simulink subsystem "BatteryHVDetailed_refsub_MultiModule"  (R2022a)
settings: Solver=VariableStepAuto  StartTime=0.0  StopTime=10.0  RelTol=1e-3
undefined symbols (not defined in the file or in its folder): batteryHV_multi_pack1, batteryHV_multi_pack2
libraries: fl_lib x139, nesl_utility x29, batteryModule_lib x12
(part 3 of 3)

== system BatteryHVDetailed_refsub_MultiModule/BatteryPack1/negPlate_B14 ==
  Conductive Heat Transfer : fl_lib/Thermal/Thermal Elements/Conductive Heat Transfer  area=batteryHV_multi_pack1.batteryCell_H*batteryHV_multi_pack1.batteryCell_W m^2  thickness=0.002 m  th_cond=0.024 W/(m*K)  T_specify=off  T_priority=None  T=0 K  T_nominal_specify=off  T_nominal_unit=K  T_nominal_value=1  Q_specify=off  Q_priority=None  Q=0 W  Q_nominal_specify=off  Q_nominal_unit=W  Q_nominal_value=1
      settings: SourceProductBaseCode=PW,SS,VE
  Conductive Heat Transfer1 : fl_lib/Thermal/Thermal Elements/Conductive Heat Transfer  area=batteryHV_multi_pack1.batteryCell_H*batteryHV_multi_pack1.batteryCell_W m^2  thickness=0.002 m  th_cond=0.024 W/(m*K)  T_specify=off  T_priority=None  T=0 K  T_nominal_specify=off  T_nominal_unit=K  T_nominal_value=1  Q_specify=off  Q_priority=None  Q=0 W  Q_nominal_specify=off  Q_nominal_unit=W  Q_nominal_value=1
      settings: SourceProductBaseCode=PW,SS,VE
  plasticPlate : fl_lib/Thermal/Thermal Elements/Thermal Mass  mass=batteryHV_multi_pack1.batteryCell_H*batteryHV_multi_pack1.batteryCell_T*batteryHV_multi_pack1.battery_N_cells*0.002*44 kg  sp_heat=400 J/kg/K  T_specify=off  T_priority=High  T=300 K  T_nominal_specify=off  T_nominal_unit=K  T_nominal_value=1  Q_specify=off  Q_priority=None  Q=0 W  Q_nominal_specify=off  Q_nominal_unit=W  Q_nominal_value=1
      settings: SourceProductBaseCode=PW,SS,VE
  amb : PMIOPort  Side=Left
  M : PMIOPort  Port=2  Side=Right
  connections:
  Conductive Heat Transfer1/LConn1 -- Conductive Heat Transfer/RConn1 -- plasticPlate/LConn1
  Conductive Heat Transfer/LConn1 -- M/RConn1
  Conductive Heat Transfer1/RConn1 -- amb/RConn1

== system BatteryHVDetailed_refsub_MultiModule/BatteryPack1/negPlate_B16 ==
  Conductive Heat Transfer : fl_lib/Thermal/Thermal Elements/Conductive Heat Transfer  area=batteryHV_multi_pack1.batteryCell_H*batteryHV_multi_pack1.batteryCell_W m^2  thickness=0.002 m  th_cond=0.024 W/(m*K)  T_specify=off  T_priority=None  T=0 K  T_nominal_specify=off  T_nominal_unit=K  T_nominal_value=1  Q_specify=off  Q_priority=None  Q=0 W  Q_nominal_specify=off  Q_nominal_unit=W  Q_nominal_value=1
      settings: SourceProductBaseCode=PW,SS,VE
  Conductive Heat Transfer1 : fl_lib/Thermal/Thermal Elements/Conductive Heat Transfer  area=batteryHV_multi_pack1.batteryCell_H*batteryHV_multi_pack1.batteryCell_W m^2  thickness=0.002 m  th_cond=0.024 W/(m*K)  T_specify=off  T_priority=None  T=0 K  T_nominal_specify=off  T_nominal_unit=K  T_nominal_value=1  Q_specify=off  Q_priority=None  Q=0 W  Q_nominal_specify=off  Q_nominal_unit=W  Q_nominal_value=1
      settings: SourceProductBaseCode=PW,SS,VE
  plasticPlate : fl_lib/Thermal/Thermal Elements/Thermal Mass  mass=batteryHV_multi_pack1.batteryCell_H*batteryHV_multi_pack1.batteryCell_T*batteryHV_multi_pack1.battery_N_cells*0.002*44 kg  sp_heat=400 J/kg/K  T_specify=off  T_priority=High  T=300 K  T_nominal_specify=off  T_nominal_unit=K  T_nominal_value=1  Q_specify=off  Q_priority=None  Q=0 W  Q_nominal_specify=off  Q_nominal_unit=W  Q_nominal_value=1
      settings: SourceProductBaseCode=PW,SS,VE
  amb : PMIOPort  Side=Left
  M : PMIOPort  Port=2  Side=Right
  connections:
  Conductive Heat Transfer1/RConn1 -- amb/RConn1
  Conductive Heat Transfer/LConn1 -- M/RConn1
  plasticPlate/LConn1 -- Conductive Heat Transfer/RConn1 -- Conductive Heat Transfer1/LConn1

== system BatteryHVDetailed_refsub_MultiModule/BatteryPack1/posPlate_B11 ==
  Conductive Heat Transfer : fl_lib/Thermal/Thermal Elements/Conductive Heat Transfer  area=batteryHV_multi_pack1.batteryCell_H*batteryHV_multi_pack1.batteryCell_W m^2  thickness=0.002 m  th_cond=0.024 W/(m*K)  T_specify=off  T_priority=None  T=0 K  T_nominal_specify=off  T_nominal_unit=K  T_nominal_value=1  Q_specify=off  Q_priority=None  Q=0 W  Q_nominal_specify=off  Q_nominal_unit=W  Q_nominal_value=1
      settings: SourceProductBaseCode=PW,SS,VE
  Conductive Heat Transfer1 : fl_lib/Thermal/Thermal Elements/Conductive Heat Transfer  area=batteryHV_multi_pack1.batteryCell_H*batteryHV_multi_pack1.batteryCell_W m^2  thickness=0.002 m  th_cond=0.024 W/(m*K)  T_specify=off  T_priority=None  T=0 K  T_nominal_specify=off  T_nominal_unit=K  T_nominal_value=1  Q_specify=off  Q_priority=None  Q=0 W  Q_nominal_specify=off  Q_nominal_unit=W  Q_nominal_value=1
      settings: SourceProductBaseCode=PW,SS,VE
  plasticPlate : fl_lib/Thermal/Thermal Elements/Thermal Mass  mass=batteryHV_multi_pack1.batteryCell_H*batteryHV_multi_pack1.batteryCell_T*batteryHV_multi_pack1.battery_N_cells*0.002*44 kg  sp_heat=400 J/kg/K  T_specify=off  T_priority=High  T=300 K  T_nominal_specify=off  T_nominal_unit=K  T_nominal_value=1  Q_specify=off  Q_priority=None  Q=0 W  Q_nominal_specify=off  Q_nominal_unit=W  Q_nominal_value=1
      settings: SourceProductBaseCode=PW,SS,VE
  amb : PMIOPort  Side=Left
  M : PMIOPort  Port=2  Side=Right
  connections:
  Conductive Heat Transfer1/RConn1 -- amb/RConn1
  Conductive Heat Transfer/LConn1 -- M/RConn1
  plasticPlate/LConn1 -- Conductive Heat Transfer/RConn1 -- Conductive Heat Transfer1/LConn1

== system BatteryHVDetailed_refsub_MultiModule/BatteryPack1/posPlate_B13 ==
  Conductive Heat Transfer : fl_lib/Thermal/Thermal Elements/Conductive Heat Transfer  area=batteryHV_multi_pack1.batteryCell_H*batteryHV_multi_pack1.batteryCell_W m^2  thickness=0.002 m  th_cond=0.024 W/(m*K)  T_specify=off  T_priority=None  T=0 K  T_nominal_specify=off  T_nominal_unit=K  T_nominal_value=1  Q_specify=off  Q_priority=None  Q=0 W  Q_nominal_specify=off  Q_nominal_unit=W  Q_nominal_value=1
      settings: SourceProductBaseCode=PW,SS,VE
  Conductive Heat Transfer1 : fl_lib/Thermal/Thermal Elements/Conductive Heat Transfer  area=batteryHV_multi_pack1.batteryCell_H*batteryHV_multi_pack1.batteryCell_W m^2  thickness=0.002 m  th_cond=0.024 W/(m*K)  T_specify=off  T_priority=None  T=0 K  T_nominal_specify=off  T_nominal_unit=K  T_nominal_value=1  Q_specify=off  Q_priority=None  Q=0 W  Q_nominal_specify=off  Q_nominal_unit=W  Q_nominal_value=1
      settings: SourceProductBaseCode=PW,SS,VE
  plasticPlate : fl_lib/Thermal/Thermal Elements/Thermal Mass  mass=batteryHV_multi_pack1.batteryCell_H*batteryHV_multi_pack1.batteryCell_T*batteryHV_multi_pack1.battery_N_cells*0.002*44 kg  sp_heat=400 J/kg/K  T_specify=off  T_priority=High  T=300 K  T_nominal_specify=off  T_nominal_unit=K  T_nominal_value=1  Q_specify=off  Q_priority=None  Q=0 W  Q_nominal_specify=off  Q_nominal_unit=W  Q_nominal_value=1
      settings: SourceProductBaseCode=PW,SS,VE
  amb : PMIOPort  Side=Left
  M : PMIOPort  Port=2  Side=Right
  connections:
  Conductive Heat Transfer1/RConn1 -- amb/RConn1
  Conductive Heat Transfer/LConn1 -- M/RConn1
  plasticPlate/LConn1 -- Conductive Heat Transfer/RConn1 -- Conductive Heat Transfer1/LConn1

== system BatteryHVDetailed_refsub_MultiModule/BatteryPack1/posPlate_B15 ==
  Conductive Heat Transfer : fl_lib/Thermal/Thermal Elements/Conductive Heat Transfer  area=batteryHV_multi_pack1.batteryCell_H*batteryHV_multi_pack1.batteryCell_W m^2  thickness=0.002 m  th_cond=0.024 W/(m*K)  T_specify=off  T_priority=None  T=0 K  T_nominal_specify=off  T_nominal_unit=K  T_nominal_value=1  Q_specify=off  Q_priority=None  Q=0 W  Q_nominal_specify=off  Q_nominal_unit=W  Q_nominal_value=1
      settings: SourceProductBaseCode=PW,SS,VE
  Conductive Heat Transfer1 : fl_lib/Thermal/Thermal Elements/Conductive Heat Transfer  area=batteryHV_multi_pack1.batteryCell_H*batteryHV_multi_pack1.batteryCell_W m^2  thickness=0.002 m  th_cond=0.024 W/(m*K)  T_specify=off  T_priority=None  T=0 K  T_nominal_specify=off  T_nominal_unit=K  T_nominal_value=1  Q_specify=off  Q_priority=None  Q=0 W  Q_nominal_specify=off  Q_nominal_unit=W  Q_nominal_value=1
      settings: SourceProductBaseCode=PW,SS,VE
  plasticPlate : fl_lib/Thermal/Thermal Elements/Thermal Mass  mass=batteryHV_multi_pack1.batteryCell_H*batteryHV_multi_pack1.batteryCell_T*batteryHV_multi_pack1.battery_N_cells*0.002*44 kg  sp_heat=400 J/kg/K  T_specify=off  T_priority=High  T=300 K  T_nominal_specify=off  T_nominal_unit=K  T_nominal_value=1  Q_specify=off  Q_priority=None  Q=0 W  Q_nominal_specify=off  Q_nominal_unit=W  Q_nominal_value=1
      settings: SourceProductBaseCode=PW,SS,VE
  amb : PMIOPort  Side=Left
  M : PMIOPort  Port=2  Side=Right
  connections:
  Conductive Heat Transfer1/LConn1 -- Conductive Heat Transfer/RConn1 -- plasticPlate/LConn1
  Conductive Heat Transfer/LConn1 -- M/RConn1
  Conductive Heat Transfer1/RConn1 -- amb/RConn1

== system BatteryHVDetailed_refsub_MultiModule/BatteryPack1/rightPlate_B15 ==
  Conductive Heat Transfer : fl_lib/Thermal/Thermal Elements/Conductive Heat Transfer  area=batteryHV_multi_pack1.batteryCell_H*batteryHV_multi_pack1.batteryCell_T*batteryHV_multi_pack1.battery_N_cells m^2  thickness=0.002 m  th_cond=0.024 W/(m*K)  T_specify=off  T_priority=None  T=0 K  T_nominal_specify=off  T_nominal_unit=K  T_nominal_value=1  Q_specify=off  Q_priority=None  Q=0 W  Q_nominal_specify=off  Q_nominal_unit=W  Q_nominal_value=1
      settings: SourceProductBaseCode=PW,SS,VE
  Conductive Heat Transfer1 : fl_lib/Thermal/Thermal Elements/Conductive Heat Transfer  area=batteryHV_multi_pack1.batteryCell_H*batteryHV_multi_pack1.batteryCell_T*batteryHV_multi_pack1.battery_N_cells m^2  thickness=0.002 m  th_cond=0.024 W/(m*K)  T_specify=off  T_priority=None  T=0 K  T_nominal_specify=off  T_nominal_unit=K  T_nominal_value=1  Q_specify=off  Q_priority=None  Q=0 W  Q_nominal_specify=off  Q_nominal_unit=W  Q_nominal_value=1
      settings: SourceProductBaseCode=PW,SS,VE
  plasticPlate : fl_lib/Thermal/Thermal Elements/Thermal Mass  mass=batteryHV_multi_pack1.batteryCell_H*batteryHV_multi_pack1.batteryCell_T*batteryHV_multi_pack1.battery_N_cells*0.002*44 kg  sp_heat=400 J/kg/K  T_specify=off  T_priority=High  T=300 K  T_nominal_specify=off  T_nominal_unit=K  T_nominal_value=1  Q_specify=off  Q_priority=None  Q=0 W  Q_nominal_specify=off  Q_nominal_unit=W  Q_nominal_value=1
      settings: SourceProductBaseCode=PW,SS,VE
  amb : PMIOPort  Side=Left
  M : PMIOPort  Port=2  Side=Right
  connections:
  Conductive Heat Transfer1/RConn1 -- amb/RConn1
  Conductive Heat Transfer/LConn1 -- M/RConn1
  plasticPlate/LConn1 -- Conductive Heat Transfer/RConn1 -- Conductive Heat Transfer1/LConn1

== system BatteryHVDetailed_refsub_MultiModule/BatteryPack1/rightPlate_B16 ==
  Conductive Heat Transfer : fl_lib/Thermal/Thermal Elements/Conductive Heat Transfer  area=batteryHV_multi_pack1.batteryCell_H*batteryHV_multi_pack1.batteryCell_T*batteryHV_multi_pack1.battery_N_cells m^2  thickness=0.002 m  th_cond=0.024 W/(m*K)  T_specify=off  T_priority=None  T=0 K  T_nominal_specify=off  T_nominal_unit=K  T_nominal_value=1  Q_specify=off  Q_priority=None  Q=0 W  Q_nominal_specify=off  Q_nominal_unit=W  Q_nominal_value=1
      settings: SourceProductBaseCode=PW,SS,VE
  Conductive Heat Transfer1 : fl_lib/Thermal/Thermal Elements/Conductive Heat Transfer  area=batteryHV_multi_pack1.batteryCell_H*batteryHV_multi_pack1.batteryCell_T*batteryHV_multi_pack1.battery_N_cells m^2  thickness=0.002 m  th_cond=0.024 W/(m*K)  T_specify=off  T_priority=None  T=0 K  T_nominal_specify=off  T_nominal_unit=K  T_nominal_value=1  Q_specify=off  Q_priority=None  Q=0 W  Q_nominal_specify=off  Q_nominal_unit=W  Q_nominal_value=1
      settings: SourceProductBaseCode=PW,SS,VE
  plasticPlate : fl_lib/Thermal/Thermal Elements/Thermal Mass  mass=batteryHV_multi_pack1.batteryCell_H*batteryHV_multi_pack1.batteryCell_T*batteryHV_multi_pack1.battery_N_cells*0.002*44 kg  sp_heat=400 J/kg/K  T_specify=off  T_priority=High  T=300 K  T_nominal_specify=off  T_nominal_unit=K  T_nominal_value=1  Q_specify=off  Q_priority=None  Q=0 W  Q_nominal_specify=off  Q_nominal_unit=W  Q_nominal_value=1
      settings: SourceProductBaseCode=PW,SS,VE
  amb : PMIOPort  Side=Left
  M : PMIOPort  Port=2  Side=Right
  connections:
  Conductive Heat Transfer1/LConn1 -- Conductive Heat Transfer/RConn1 -- plasticPlate/LConn1
  Conductive Heat Transfer/LConn1 -- M/RConn1
  Conductive Heat Transfer1/RConn1 -- amb/RConn1

== system BatteryHVDetailed_refsub_MultiModule/BatteryPack2/air gap 2-1 ==
  Conductive Heat Transfer : fl_lib/Thermal/Thermal Elements/Conductive Heat Transfer  area=batteryHV_multi_pack1.batteryCell_T*batteryHV_multi_pack1.battery_N_cells*batteryHV_multi_pack1.batteryCell_H m^2  thickness=0.002 m  th_cond=0.024 W/(m*K)  T_specify=off  T_priority=None  T=0 K  T_nominal_specify=off  T_nominal_unit=K  T_nominal_value=1  Q_specify=off  Q_priority=None  Q=0 W  Q_nominal_specify=off  Q_nominal_unit=W  Q_nominal_value=1
      settings: SourceProductBaseCode=PW,SS,VE
  Conductive Heat Transfer1 : fl_lib/Thermal/Thermal Elements/Conductive Heat Transfer  area=batteryHV_multi_pack1.batteryCell_H*batteryHV_multi_pack1.batteryCell_H m^2  thickness=0.002 m  th_cond=0.024 W/(m*K)  T_specify=off  T_priority=None  T=0 K  T_nominal_specify=off  T_nominal_unit=K  T_nominal_value=1  Q_specify=off  Q_priority=None  Q=0 W  Q_nominal_specify=off  Q_nominal_unit=W  Q_nominal_value=1
      settings: SourceProductBaseCode=PW,SS,VE
  air mass : fl_lib/Thermal/Thermal Elements/Thermal Mass  mass=batteryHV_multi_pack1.batteryCell_H*batteryHV_multi_pack1.batteryCell_T*batteryHV_multi_pack1.battery_N_cells*0.002*1.28 kg  sp_heat=1000 J/kg/K  T_specify=off  T_priority=High  T=300 K  T_nominal_specify=off  T_nominal_unit=K  T_nominal_value=1  Q_specify=off  Q_priority=None  Q=0 W  Q_nominal_specify=off  Q_nominal_unit=W  Q_nominal_value=1
      settings: SourceProductBaseCode=PW,SS,VE
  M2 : PMIOPort  Side=Left
  M1 : PMIOPort  Port=2  Side=Right
  connections:
  Conductive Heat Transfer1/LConn1 -- Conductive Heat Transfer/RConn1 -- air mass/LConn1
  Conductive Heat Transfer1/RConn1 -- M1/RConn1
  Conductive Heat Transfer/LConn1 -- M2/RConn1

== system BatteryHVDetailed_refsub_MultiModule/BatteryPack2/air gap 3-2 ==
  Conductive Heat Transfer : fl_lib/Thermal/Thermal Elements/Conductive Heat Transfer  area=batteryHV_multi_pack1.batteryCell_T*batteryHV_multi_pack1.battery_N_cells*batteryHV_multi_pack1.batteryCell_H m^2  thickness=0.002 m  th_cond=0.024 W/(m*K)  T_specify=off  T_priority=None  T=0 K  T_nominal_specify=off  T_nominal_unit=K  T_nominal_value=1  Q_specify=off  Q_priority=None  Q=0 W  Q_nominal_specify=off  Q_nominal_unit=W  Q_nominal_value=1
      settings: SourceProductBaseCode=PW,SS,VE
  Conductive Heat Transfer1 : fl_lib/Thermal/Thermal Elements/Conductive Heat Transfer  area=batteryHV_multi_pack1.batteryCell_H*batteryHV_multi_pack1.batteryCell_H m^2  thickness=0.002 m  th_cond=0.024 W/(m*K)  T_specify=off  T_priority=None  T=0 K  T_nominal_specify=off  T_nominal_unit=K  T_nominal_value=1  Q_specify=off  Q_priority=None  Q=0 W  Q_nominal_specify=off  Q_nominal_unit=W  Q_nominal_value=1
      settings: SourceProductBaseCode=PW,SS,VE
  air mass : fl_lib/Thermal/Thermal Elements/Thermal Mass  mass=batteryHV_multi_pack1.batteryCell_H*batteryHV_multi_pack1.batteryCell_T*batteryHV_multi_pack1.battery_N_cells*0.002*1.28 kg  sp_heat=1000 J/kg/K  T_specify=off  T_priority=High  T=300 K  T_nominal_specify=off  T_nominal_unit=K  T_nominal_value=1  Q_specify=off  Q_priority=None  Q=0 W  Q_nominal_specify=off  Q_nominal_unit=W  Q_nominal_value=1
      settings: SourceProductBaseCode=PW,SS,VE
  M3 : PMIOPort  Side=Left
  M2 : PMIOPort  Port=2  Side=Right
  connections:
  Conductive Heat Transfer/LConn1 -- M3/RConn1
  Conductive Heat Transfer1/RConn1 -- M2/RConn1
  air mass/LConn1 -- Conductive Heat Transfer/RConn1 -- Conductive Heat Transfer1/LConn1

== system BatteryHVDetailed_refsub_MultiModule/BatteryPack2/air gap 4-3 ==
  Conductive Heat Transfer : fl_lib/Thermal/Thermal Elements/Conductive Heat Transfer  area=batteryHV_multi_pack1.batteryCell_T*batteryHV_multi_pack1.battery_N_cells*batteryHV_multi_pack1.batteryCell_H m^2  thickness=0.002 m  th_cond=0.024 W/(m*K)  T_specify=off  T_priority=None  T=0 K  T_nominal_specify=off  T_nominal_unit=K  T_nominal_value=1  Q_specify=off  Q_priority=None  Q=0 W  Q_nominal_specify=off  Q_nominal_unit=W  Q_nominal_value=1
      settings: SourceProductBaseCode=PW,SS,VE
  Conductive Heat Transfer1 : fl_lib/Thermal/Thermal Elements/Conductive Heat Transfer  area=batteryHV_multi_pack1.batteryCell_H*batteryHV_multi_pack1.batteryCell_H m^2  thickness=0.002 m  th_cond=0.024 W/(m*K)  T_specify=off  T_priority=None  T=0 K  T_nominal_specify=off  T_nominal_unit=K  T_nominal_value=1  Q_specify=off  Q_priority=None  Q=0 W  Q_nominal_specify=off  Q_nominal_unit=W  Q_nominal_value=1
      settings: SourceProductBaseCode=PW,SS,VE
  air mass : fl_lib/Thermal/Thermal Elements/Thermal Mass  mass=batteryHV_multi_pack1.batteryCell_H*batteryHV_multi_pack1.batteryCell_T*batteryHV_multi_pack1.battery_N_cells*0.002*1.28 kg  sp_heat=1000 J/kg/K  T_specify=off  T_priority=High  T=300 K  T_nominal_specify=off  T_nominal_unit=K  T_nominal_value=1  Q_specify=off  Q_priority=None  Q=0 W  Q_nominal_specify=off  Q_nominal_unit=W  Q_nominal_value=1
      settings: SourceProductBaseCode=PW,SS,VE
  M4 : PMIOPort  Side=Left
  M3 : PMIOPort  Port=2  Side=Right
  connections:
  Conductive Heat Transfer1/LConn1 -- Conductive Heat Transfer/RConn1 -- air mass/LConn1
  Conductive Heat Transfer1/RConn1 -- M3/RConn1
  Conductive Heat Transfer/LConn1 -- M4/RConn1

== system BatteryHVDetailed_refsub_MultiModule/BatteryPack2/air gap 5-4 ==
  Conductive Heat Transfer : fl_lib/Thermal/Thermal Elements/Conductive Heat Transfer  area=batteryHV_multi_pack1.batteryCell_T*batteryHV_multi_pack1.battery_N_cells*batteryHV_multi_pack1.batteryCell_H m^2  thickness=0.002 m  th_cond=0.024 W/(m*K)  T_specify=off  T_priority=None  T=0 K  T_nominal_specify=off  T_nominal_unit=K  T_nominal_value=1  Q_specify=off  Q_priority=None  Q=0 W  Q_nominal_specify=off  Q_nominal_unit=W  Q_nominal_value=1
      settings: SourceProductBaseCode=PW,SS,VE
  Conductive Heat Transfer1 : fl_lib/Thermal/Thermal Elements/Conductive Heat Transfer  area=batteryHV_multi_pack1.batteryCell_H*batteryHV_multi_pack1.batteryCell_H m^2  thickness=0.002 m  th_cond=0.024 W/(m*K)  T_specify=off  T_priority=None  T=0 K  T_nominal_specify=off  T_nominal_unit=K  T_nominal_value=1  Q_specify=off  Q_priority=None  Q=0 W  Q_nominal_specify=off  Q_nominal_unit=W  Q_nominal_value=1
      settings: SourceProductBaseCode=PW,SS,VE
  air mass : fl_lib/Thermal/Thermal Elements/Thermal Mass  mass=batteryHV_multi_pack1.batteryCell_H*batteryHV_multi_pack1.batteryCell_T*batteryHV_multi_pack1.battery_N_cells*0.002*1.28 kg  sp_heat=1000 J/kg/K  T_specify=off  T_priority=High  T=300 K  T_nominal_specify=off  T_nominal_unit=K  T_nominal_value=1  Q_specify=off  Q_priority=None  Q=0 W  Q_nominal_specify=off  Q_nominal_unit=W  Q_nominal_value=1
      settings: SourceProductBaseCode=PW,SS,VE
  M5 : PMIOPort  Side=Left
  M4 : PMIOPort  Port=2  Side=Right
  connections:
  Conductive Heat Transfer/LConn1 -- M5/RConn1
  Conductive Heat Transfer1/RConn1 -- M4/RConn1
  air mass/LConn1 -- Conductive Heat Transfer/RConn1 -- Conductive Heat Transfer1/LConn1

== system BatteryHVDetailed_refsub_MultiModule/BatteryPack2/air gap 5-6 ==
  Conductive Heat Transfer : fl_lib/Thermal/Thermal Elements/Conductive Heat Transfer  area=batteryHV_multi_pack2.batteryCell_T*batteryHV_multi_pack2.battery_N_cells*batteryHV_multi_pack2.batteryCell_W m^2  thickness=0.002 m  th_cond=0.024 W/(m*K)  T_specify=off  T_priority=None  T=0 K  T_nominal_specify=off  T_nominal_unit=K  T_nominal_value=1  Q_specify=off  Q_priority=None  Q=0 W  Q_nominal_specify=off  Q_nominal_unit=W  Q_nominal_value=1
      settings: SourceProductBaseCode=PW,SS,VE
  Conductive Heat Transfer1 : fl_lib/Thermal/Thermal Elements/Conductive Heat Transfer  area=batteryHV_multi_pack2.batteryCell_H*batteryHV_multi_pack2.batteryCell_W m^2  thickness=0.002 m  th_cond=0.024 W/(m*K)  T_specify=off  T_priority=None  T=0 K  T_nominal_specify=off  T_nominal_unit=K  T_nominal_value=1  Q_specify=off  Q_priority=None  Q=0 W  Q_nominal_specify=off  Q_nominal_unit=W  Q_nominal_value=1
      settings: SourceProductBaseCode=PW,SS,VE
  air mass : fl_lib/Thermal/Thermal Elements/Thermal Mass  mass=batteryHV_multi_pack2.batteryCell_W*batteryHV_multi_pack2.batteryCell_T*batteryHV_multi_pack2.battery_N_cells*0.002*1.28 kg  sp_heat=1000 J/kg/K  T_specify=off  T_priority=High  T=300 K  T_nominal_specify=off  T_nominal_unit=K  T_nominal_value=1  Q_specify=off  Q_priority=None  Q=0 W  Q_nominal_specify=off  Q_nominal_unit=W  Q_nominal_value=1
      settings: SourceProductBaseCode=PW,SS,VE
  M5 : PMIOPort  Side=Left
  M6 : PMIOPort  Port=2  Side=Right
  connections:
  Conductive Heat Transfer/LConn1 -- M5/RConn1
  Conductive Heat Transfer1/RConn1 -- M6/RConn1
  air mass/LConn1 -- Conductive Heat Transfer/RConn1 -- Conductive Heat Transfer1/LConn1

== system BatteryHVDetailed_refsub_MultiModule/BatteryPack2/leftPlate_B11 ==
  Conductive Heat Transfer : fl_lib/Thermal/Thermal Elements/Conductive Heat Transfer  area=batteryHV_multi_pack2.batteryCell_H*batteryHV_multi_pack2.batteryCell_T*batteryHV_multi_pack2.battery_N_cells m^2  thickness=0.002 m  th_cond=0.024 W/(m*K)  T_specify=off  T_priority=None  T=0 K  T_nominal_specify=off  T_nominal_unit=K  T_nominal_value=1  Q_specify=off  Q_priority=None  Q=0 W  Q_nominal_specify=off  Q_nominal_unit=W  Q_nominal_value=1
      settings: SourceProductBaseCode=PW,SS,VE
  Conductive Heat Transfer1 : fl_lib/Thermal/Thermal Elements/Conductive Heat Transfer  area=batteryHV_multi_pack2.batteryCell_H*batteryHV_multi_pack2.batteryCell_T*batteryHV_multi_pack2.battery_N_cells m^2  thickness=0.002 m  th_cond=0.024 W/(m*K)  T_specify=off  T_priority=None  T=0 K  T_nominal_specify=off  T_nominal_unit=K  T_nominal_value=1  Q_specify=off  Q_priority=None  Q=0 W  Q_nominal_specify=off  Q_nominal_unit=W  Q_nominal_value=1
      settings: SourceProductBaseCode=PW,SS,VE
  plasticPlate : fl_lib/Thermal/Thermal Elements/Thermal Mass  mass=batteryHV_multi_pack2.batteryCell_H*batteryHV_multi_pack2.batteryCell_T*batteryHV_multi_pack2.battery_N_cells*0.002*44 kg  sp_heat=400 J/kg/K  T_specify=off  T_priority=High  T=300 K  T_nominal_specify=off  T_nominal_unit=K  T_nominal_value=1  Q_specify=off  Q_priority=None  Q=0 W  Q_nominal_specify=off  Q_nominal_unit=W  Q_nominal_value=1
      settings: SourceProductBaseCode=PW,SS,VE
  amb : PMIOPort  Side=Left
  M : PMIOPort  Port=2  Side=Right
  connections:
  Conductive Heat Transfer1/LConn1 -- Conductive Heat Transfer/RConn1 -- plasticPlate/LConn1
  Conductive Heat Transfer/LConn1 -- M/RConn1
  Conductive Heat Transfer1/RConn1 -- amb/RConn1

== system BatteryHVDetailed_refsub_MultiModule/BatteryPack2/leftPlate_B16 ==
  Conductive Heat Transfer : fl_lib/Thermal/Thermal Elements/Conductive Heat Transfer  area=batteryHV_multi_pack2.batteryCell_H*batteryHV_multi_pack2.batteryCell_T*batteryHV_multi_pack2.battery_N_cells m^2  thickness=0.002 m  th_cond=0.024 W/(m*K)  T_specify=off  T_priority=None  T=0 K  T_nominal_specify=off  T_nominal_unit=K  T_nominal_value=1  Q_specify=off  Q_priority=None  Q=0 W  Q_nominal_specify=off  Q_nominal_unit=W  Q_nominal_value=1
      settings: SourceProductBaseCode=PW,SS,VE
  Conductive Heat Transfer1 : fl_lib/Thermal/Thermal Elements/Conductive Heat Transfer  area=batteryHV_multi_pack2.batteryCell_H*batteryHV_multi_pack2.batteryCell_T*batteryHV_multi_pack2.battery_N_cells m^2  thickness=0.002 m  th_cond=0.024 W/(m*K)  T_specify=off  T_priority=None  T=0 K  T_nominal_specify=off  T_nominal_unit=K  T_nominal_value=1  Q_specify=off  Q_priority=None  Q=0 W  Q_nominal_specify=off  Q_nominal_unit=W  Q_nominal_value=1
      settings: SourceProductBaseCode=PW,SS,VE
  plasticPlate : fl_lib/Thermal/Thermal Elements/Thermal Mass  mass=batteryHV_multi_pack2.batteryCell_H*batteryHV_multi_pack2.batteryCell_T*batteryHV_multi_pack2.battery_N_cells*0.002*44 kg  sp_heat=400 J/kg/K  T_specify=off  T_priority=High  T=300 K  T_nominal_specify=off  T_nominal_unit=K  T_nominal_value=1  Q_specify=off  Q_priority=None  Q=0 W  Q_nominal_specify=off  Q_nominal_unit=W  Q_nominal_value=1
      settings: SourceProductBaseCode=PW,SS,VE
  amb : PMIOPort  Side=Left
  M : PMIOPort  Port=2  Side=Right
  connections:
  Conductive Heat Transfer1/LConn1 -- Conductive Heat Transfer/RConn1 -- plasticPlate/LConn1
  Conductive Heat Transfer/LConn1 -- M/RConn1
  Conductive Heat Transfer1/RConn1 -- amb/RConn1

== system BatteryHVDetailed_refsub_MultiModule/BatteryPack2/negPlate_B12 ==
  Conductive Heat Transfer : fl_lib/Thermal/Thermal Elements/Conductive Heat Transfer  area=batteryHV_multi_pack2.batteryCell_H*batteryHV_multi_pack2.batteryCell_W m^2  thickness=0.002 m  th_cond=0.024 W/(m*K)  T_specify=off  T_priority=None  T=0 K  T_nominal_specify=off  T_nominal_unit=K  T_nominal_value=1  Q_specify=off  Q_priority=None  Q=0 W  Q_nominal_specify=off  Q_nominal_unit=W  Q_nominal_value=1
      settings: SourceProductBaseCode=PW,SS,VE
  Conductive Heat Transfer1 : fl_lib/Thermal/Thermal Elements/Conductive Heat Transfer  area=batteryHV_multi_pack2.batteryCell_H*batteryHV_multi_pack2.batteryCell_W m^2  thickness=0.002 m  th_cond=0.024 W/(m*K)  T_specify=off  T_priority=None  T=0 K  T_nominal_specify=off  T_nominal_unit=K  T_nominal_value=1  Q_specify=off  Q_priority=None  Q=0 W  Q_nominal_specify=off  Q_nominal_unit=W  Q_nominal_value=1
      settings: SourceProductBaseCode=PW,SS,VE
  plasticPlate : fl_lib/Thermal/Thermal Elements/Thermal Mass  mass=batteryHV_multi_pack2.batteryCell_H*batteryHV_multi_pack2.batteryCell_T*batteryHV_multi_pack2.battery_N_cells*0.002*44 kg  sp_heat=400 J/kg/K  T_specify=off  T_priority=High  T=300 K  T_nominal_specify=off  T_nominal_unit=K  T_nominal_value=1  Q_specify=off  Q_priority=None  Q=0 W  Q_nominal_specify=off  Q_nominal_unit=W  Q_nominal_value=1
      settings: SourceProductBaseCode=PW,SS,VE
  amb : PMIOPort  Side=Left
  M : PMIOPort  Port=2  Side=Right
  connections:
  Conductive Heat Transfer1/RConn1 -- amb/RConn1
  Conductive Heat Transfer/LConn1 -- M/RConn1
  plasticPlate/LConn1 -- Conductive Heat Transfer/RConn1 -- Conductive Heat Transfer1/LConn1

== system BatteryHVDetailed_refsub_MultiModule/BatteryPack2/negPlate_B14 ==
  Conductive Heat Transfer : fl_lib/Thermal/Thermal Elements/Conductive Heat Transfer  area=batteryHV_multi_pack2.batteryCell_H*batteryHV_multi_pack2.batteryCell_W m^2  thickness=0.002 m  th_cond=0.024 W/(m*K)  T_specify=off  T_priority=None  T=0 K  T_nominal_specify=off  T_nominal_unit=K  T_nominal_value=1  Q_specify=off  Q_priority=None  Q=0 W  Q_nominal_specify=off  Q_nominal_unit=W  Q_nominal_value=1
      settings: SourceProductBaseCode=PW,SS,VE
  Conductive Heat Transfer1 : fl_lib/Thermal/Thermal Elements/Conductive Heat Transfer  area=batteryHV_multi_pack2.batteryCell_H*batteryHV_multi_pack2.batteryCell_W m^2  thickness=0.002 m  th_cond=0.024 W/(m*K)  T_specify=off  T_priority=None  T=0 K  T_nominal_specify=off  T_nominal_unit=K  T_nominal_value=1  Q_specify=off  Q_priority=None  Q=0 W  Q_nominal_specify=off  Q_nominal_unit=W  Q_nominal_value=1
      settings: SourceProductBaseCode=PW,SS,VE
  plasticPlate : fl_lib/Thermal/Thermal Elements/Thermal Mass  mass=batteryHV_multi_pack2.batteryCell_H*batteryHV_multi_pack2.batteryCell_T*batteryHV_multi_pack2.battery_N_cells*0.002*44 kg  sp_heat=400 J/kg/K  T_specify=off  T_priority=High  T=300 K  T_nominal_specify=off  T_nominal_unit=K  T_nominal_value=1  Q_specify=off  Q_priority=None  Q=0 W  Q_nominal_specify=off  Q_nominal_unit=W  Q_nominal_value=1
      settings: SourceProductBaseCode=PW,SS,VE
  amb : PMIOPort  Side=Left
  M : PMIOPort  Port=2  Side=Right
  connections:
  Conductive Heat Transfer1/RConn1 -- amb/RConn1
  Conductive Heat Transfer/LConn1 -- M/RConn1
  plasticPlate/LConn1 -- Conductive Heat Transfer/RConn1 -- Conductive Heat Transfer1/LConn1

== system BatteryHVDetailed_refsub_MultiModule/BatteryPack2/negPlate_B16 ==
  Conductive Heat Transfer : fl_lib/Thermal/Thermal Elements/Conductive Heat Transfer  area=batteryHV_multi_pack2.batteryCell_H*batteryHV_multi_pack2.batteryCell_W m^2  thickness=0.002 m  th_cond=0.024 W/(m*K)  T_specify=off  T_priority=None  T=0 K  T_nominal_specify=off  T_nominal_unit=K  T_nominal_value=1  Q_specify=off  Q_priority=None  Q=0 W  Q_nominal_specify=off  Q_nominal_unit=W  Q_nominal_value=1
      settings: SourceProductBaseCode=PW,SS,VE
  Conductive Heat Transfer1 : fl_lib/Thermal/Thermal Elements/Conductive Heat Transfer  area=batteryHV_multi_pack2.batteryCell_H*batteryHV_multi_pack2.batteryCell_W m^2  thickness=0.002 m  th_cond=0.024 W/(m*K)  T_specify=off  T_priority=None  T=0 K  T_nominal_specify=off  T_nominal_unit=K  T_nominal_value=1  Q_specify=off  Q_priority=None  Q=0 W  Q_nominal_specify=off  Q_nominal_unit=W  Q_nominal_value=1
      settings: SourceProductBaseCode=PW,SS,VE
  plasticPlate : fl_lib/Thermal/Thermal Elements/Thermal Mass  mass=batteryHV_multi_pack2.batteryCell_H*batteryHV_multi_pack2.batteryCell_T*batteryHV_multi_pack2.battery_N_cells*0.002*44 kg  sp_heat=400 J/kg/K  T_specify=off  T_priority=High  T=300 K  T_nominal_specify=off  T_nominal_unit=K  T_nominal_value=1  Q_specify=off  Q_priority=None  Q=0 W  Q_nominal_specify=off  Q_nominal_unit=W  Q_nominal_value=1
      settings: SourceProductBaseCode=PW,SS,VE
  amb : PMIOPort  Side=Left
  M : PMIOPort  Port=2  Side=Right
  connections:
  Conductive Heat Transfer1/LConn1 -- Conductive Heat Transfer/RConn1 -- plasticPlate/LConn1
  Conductive Heat Transfer/LConn1 -- M/RConn1
  Conductive Heat Transfer1/RConn1 -- amb/RConn1

== system BatteryHVDetailed_refsub_MultiModule/BatteryPack2/posPlate_B11 ==
  Conductive Heat Transfer : fl_lib/Thermal/Thermal Elements/Conductive Heat Transfer  area=batteryHV_multi_pack2.batteryCell_H*batteryHV_multi_pack2.batteryCell_W m^2  thickness=0.002 m  th_cond=0.024 W/(m*K)  T_specify=off  T_priority=None  T=0 K  T_nominal_specify=off  T_nominal_unit=K  T_nominal_value=1  Q_specify=off  Q_priority=None  Q=0 W  Q_nominal_specify=off  Q_nominal_unit=W  Q_nominal_value=1
      settings: SourceProductBaseCode=PW,SS,VE
  Conductive Heat Transfer1 : fl_lib/Thermal/Thermal Elements/Conductive Heat Transfer  area=batteryHV_multi_pack2.batteryCell_H*batteryHV_multi_pack2.batteryCell_W m^2  thickness=0.002 m  th_cond=0.024 W/(m*K)  T_specify=off  T_priority=None  T=0 K  T_nominal_specify=off  T_nominal_unit=K  T_nominal_value=1  Q_specify=off  Q_priority=None  Q=0 W  Q_nominal_specify=off  Q_nominal_unit=W  Q_nominal_value=1
      settings: SourceProductBaseCode=PW,SS,VE
  plasticPlate : fl_lib/Thermal/Thermal Elements/Thermal Mass  mass=batteryHV_multi_pack2.batteryCell_H*batteryHV_multi_pack2.batteryCell_T*batteryHV_multi_pack2.battery_N_cells*0.002*44 kg  sp_heat=400 J/kg/K  T_specify=off  T_priority=High  T=300 K  T_nominal_specify=off  T_nominal_unit=K  T_nominal_value=1  Q_specify=off  Q_priority=None  Q=0 W  Q_nominal_specify=off  Q_nominal_unit=W  Q_nominal_value=1
      settings: SourceProductBaseCode=PW,SS,VE
  amb : PMIOPort  Side=Left
  M : PMIOPort  Port=2  Side=Right
  connections:
  Conductive Heat Transfer1/LConn1 -- Conductive Heat Transfer/RConn1 -- plasticPlate/LConn1
  Conductive Heat Transfer/LConn1 -- M/RConn1
  Conductive Heat Transfer1/RConn1 -- amb/RConn1

== system BatteryHVDetailed_refsub_MultiModule/BatteryPack2/posPlate_B13 ==
  Conductive Heat Transfer : fl_lib/Thermal/Thermal Elements/Conductive Heat Transfer  area=batteryHV_multi_pack2.batteryCell_H*batteryHV_multi_pack2.batteryCell_W m^2  thickness=0.002 m  th_cond=0.024 W/(m*K)  T_specify=off  T_priority=None  T=0 K  T_nominal_specify=off  T_nominal_unit=K  T_nominal_value=1  Q_specify=off  Q_priority=None  Q=0 W  Q_nominal_specify=off  Q_nominal_unit=W  Q_nominal_value=1
      settings: SourceProductBaseCode=PW,SS,VE
  Conductive Heat Transfer1 : fl_lib/Thermal/Thermal Elements/Conductive Heat Transfer  area=batteryHV_multi_pack2.batteryCell_H*batteryHV_multi_pack2.batteryCell_W m^2  thickness=0.002 m  th_cond=0.024 W/(m*K)  T_specify=off  T_priority=None  T=0 K  T_nominal_specify=off  T_nominal_unit=K  T_nominal_value=1  Q_specify=off  Q_priority=None  Q=0 W  Q_nominal_specify=off  Q_nominal_unit=W  Q_nominal_value=1
      settings: SourceProductBaseCode=PW,SS,VE
  plasticPlate : fl_lib/Thermal/Thermal Elements/Thermal Mass  mass=batteryHV_multi_pack2.batteryCell_H*batteryHV_multi_pack2.batteryCell_T*batteryHV_multi_pack2.battery_N_cells*0.002*44 kg  sp_heat=400 J/kg/K  T_specify=off  T_priority=High  T=300 K  T_nominal_specify=off  T_nominal_unit=K  T_nominal_value=1  Q_specify=off  Q_priority=None  Q=0 W  Q_nominal_specify=off  Q_nominal_unit=W  Q_nominal_value=1
      settings: SourceProductBaseCode=PW,SS,VE
  amb : PMIOPort  Side=Left
  M : PMIOPort  Port=2  Side=Right
  connections:
  Conductive Heat Transfer1/LConn1 -- Conductive Heat Transfer/RConn1 -- plasticPlate/LConn1
  Conductive Heat Transfer/LConn1 -- M/RConn1
  Conductive Heat Transfer1/RConn1 -- amb/RConn1

== system BatteryHVDetailed_refsub_MultiModule/BatteryPack2/posPlate_B15 ==
  Conductive Heat Transfer : fl_lib/Thermal/Thermal Elements/Conductive Heat Transfer  area=batteryHV_multi_pack2.batteryCell_H*batteryHV_multi_pack2.batteryCell_W m^2  thickness=0.002 m  th_cond=0.024 W/(m*K)  T_specify=off  T_priority=None  T=0 K  T_nominal_specify=off  T_nominal_unit=K  T_nominal_value=1  Q_specify=off  Q_priority=None  Q=0 W  Q_nominal_specify=off  Q_nominal_unit=W  Q_nominal_value=1
      settings: SourceProductBaseCode=PW,SS,VE
  Conductive Heat Transfer1 : fl_lib/Thermal/Thermal Elements/Conductive Heat Transfer  area=batteryHV_multi_pack2.batteryCell_H*batteryHV_multi_pack2.batteryCell_W m^2  thickness=0.002 m  th_cond=0.024 W/(m*K)  T_specify=off  T_priority=None  T=0 K  T_nominal_specify=off  T_nominal_unit=K  T_nominal_value=1  Q_specify=off  Q_priority=None  Q=0 W  Q_nominal_specify=off  Q_nominal_unit=W  Q_nominal_value=1
      settings: SourceProductBaseCode=PW,SS,VE
  plasticPlate : fl_lib/Thermal/Thermal Elements/Thermal Mass  mass=batteryHV_multi_pack2.batteryCell_H*batteryHV_multi_pack2.batteryCell_T*batteryHV_multi_pack2.battery_N_cells*0.002*44 kg  sp_heat=400 J/kg/K  T_specify=off  T_priority=High  T=300 K  T_nominal_specify=off  T_nominal_unit=K  T_nominal_value=1  Q_specify=off  Q_priority=None  Q=0 W  Q_nominal_specify=off  Q_nominal_unit=W  Q_nominal_value=1
      settings: SourceProductBaseCode=PW,SS,VE
  amb : PMIOPort  Side=Left
  M : PMIOPort  Port=2  Side=Right
  connections:
  Conductive Heat Transfer1/RConn1 -- amb/RConn1
  Conductive Heat Transfer/LConn1 -- M/RConn1
  plasticPlate/LConn1 -- Conductive Heat Transfer/RConn1 -- Conductive Heat Transfer1/LConn1

== system BatteryHVDetailed_refsub_MultiModule/BatteryPack2/rightPlate_B15 ==
  Conductive Heat Transfer : fl_lib/Thermal/Thermal Elements/Conductive Heat Transfer  area=batteryHV_multi_pack2.batteryCell_H*batteryHV_multi_pack2.batteryCell_T*batteryHV_multi_pack2.battery_N_cells m^2  thickness=0.002 m  th_cond=0.024 W/(m*K)  T_specify=off  T_priority=None  T=0 K  T_nominal_specify=off  T_nominal_unit=K  T_nominal_value=1  Q_specify=off  Q_priority=None  Q=0 W  Q_nominal_specify=off  Q_nominal_unit=W  Q_nominal_value=1
      settings: SourceProductBaseCode=PW,SS,VE
  Conductive Heat Transfer1 : fl_lib/Thermal/Thermal Elements/Conductive Heat Transfer  area=batteryHV_multi_pack2.batteryCell_H*batteryHV_multi_pack2.batteryCell_T*batteryHV_multi_pack2.battery_N_cells m^2  thickness=0.002 m  th_cond=0.024 W/(m*K)  T_specify=off  T_priority=None  T=0 K  T_nominal_specify=off  T_nominal_unit=K  T_nominal_value=1  Q_specify=off  Q_priority=None  Q=0 W  Q_nominal_specify=off  Q_nominal_unit=W  Q_nominal_value=1
      settings: SourceProductBaseCode=PW,SS,VE
  plasticPlate : fl_lib/Thermal/Thermal Elements/Thermal Mass  mass=batteryHV_multi_pack2.batteryCell_H*batteryHV_multi_pack2.batteryCell_T*batteryHV_multi_pack2.battery_N_cells*0.002*44 kg  sp_heat=400 J/kg/K  T_specify=off  T_priority=High  T=300 K  T_nominal_specify=off  T_nominal_unit=K  T_nominal_value=1  Q_specify=off  Q_priority=None  Q=0 W  Q_nominal_specify=off  Q_nominal_unit=W  Q_nominal_value=1
      settings: SourceProductBaseCode=PW,SS,VE
  amb : PMIOPort  Side=Left
  M : PMIOPort  Port=2  Side=Right
  connections:
  Conductive Heat Transfer1/LConn1 -- Conductive Heat Transfer/RConn1 -- plasticPlate/LConn1
  Conductive Heat Transfer/LConn1 -- M/RConn1
  Conductive Heat Transfer1/RConn1 -- amb/RConn1

== system BatteryHVDetailed_refsub_MultiModule/BatteryPack2/rightPlate_B16 ==
  Conductive Heat Transfer : fl_lib/Thermal/Thermal Elements/Conductive Heat Transfer  area=batteryHV_multi_pack2.batteryCell_H*batteryHV_multi_pack2.batteryCell_T*batteryHV_multi_pack2.battery_N_cells m^2  thickness=0.002 m  th_cond=0.024 W/(m*K)  T_specify=off  T_priority=None  T=0 K  T_nominal_specify=off  T_nominal_unit=K  T_nominal_value=1  Q_specify=off  Q_priority=None  Q=0 W  Q_nominal_specify=off  Q_nominal_unit=W  Q_nominal_value=1
      settings: SourceProductBaseCode=PW,SS,VE
  Conductive Heat Transfer1 : fl_lib/Thermal/Thermal Elements/Conductive Heat Transfer  area=batteryHV_multi_pack2.batteryCell_H*batteryHV_multi_pack2.batteryCell_T*batteryHV_multi_pack2.battery_N_cells m^2  thickness=0.002 m  th_cond=0.024 W/(m*K)  T_specify=off  T_priority=None  T=0 K  T_nominal_specify=off  T_nominal_unit=K  T_nominal_value=1  Q_specify=off  Q_priority=None  Q=0 W  Q_nominal_specify=off  Q_nominal_unit=W  Q_nominal_value=1
      settings: SourceProductBaseCode=PW,SS,VE
  plasticPlate : fl_lib/Thermal/Thermal Elements/Thermal Mass  mass=batteryHV_multi_pack2.batteryCell_H*batteryHV_multi_pack2.batteryCell_T*batteryHV_multi_pack2.battery_N_cells*0.002*44 kg  sp_heat=400 J/kg/K  T_specify=off  T_priority=High  T=300 K  T_nominal_specify=off  T_nominal_unit=K  T_nominal_value=1  Q_specify=off  Q_priority=None  Q=0 W  Q_nominal_specify=off  Q_nominal_unit=W  Q_nominal_value=1
      settings: SourceProductBaseCode=PW,SS,VE
  amb : PMIOPort  Side=Left
  M : PMIOPort  Port=2  Side=Right
  connections:
  Conductive Heat Transfer1/RConn1 -- amb/RConn1
  Conductive Heat Transfer/LConn1 -- M/RConn1
  plasticPlate/LConn1 -- Conductive Heat Transfer/RConn1 -- Conductive Heat Transfer1/LConn1
